simulink model "gm_tutorial1_1_mq"  (R2020b)
settings: Solver=FixedStepDiscrete  StartTime=0.0  StopTime=simulation_stop_time  RelTol=1e-3
undefined symbols (not defined in the file or in its folder): sample_time
libraries: simulink x1, modelsimlib x1
settings Model: Creator=yixingli  LastModifiedBy=harsh
settings DataIOCC: LimitDataPoints=on  SaveOutput=off  SignalLogging=off  SaveTime=off
settings OptimizationCC: BlockReduction=off  ConditionallyExecuteInputs=off  DefaultParameterBehavior=Inlined  ExpressionDepthLimit=2147483647  LifeSpan=inf
settings DebuggingCC: AlgebraicLoopMsg=error  UnderspecifiedInitializationDetection=Classic  MergeDetectMultiDrivingBlocksExec=none  InheritedTsInSrcMsg=none  SingleTaskRateTransMsg=error  ParameterPrecisionLossMsg=none  AllowSymbolicDim=off  StateNameClashWarn=warning  StrictBusMsg=ErrorOnBusTreatedAsVector  SFUnexpectedBacktrackingDiag=warning  SFNoUnconditionalDefaultTransitionDiag=warning  SFExecutionAtInitializationDiag=none  ArithmeticOperatorsInVariantConditions=warning
settings HardwareCC: ProdBitPerPointer=32  ProdBitPerSizeT=32  ProdBitPerPtrDiffT=32  ProdLargestAtomicFloat=None  ProdIntDivRoundTo=Undefined  ProdEndianess=Unspecified  ProdWordSize=32  ProdHWDeviceType=ASIC/FPGA->ASIC/FPGA  ProdEqTarget=off
settings SFSimCC: SimUseLocalCustomCode=off  CustomCodeUndefinedFunction=UseInterfaceOnly
settings RTWCC: RTWUseLocalCustomCode=off
settings CodeAppCC: StateflowObjectComments=on
settings GRTTargetCC: TargetLangStandard=C89/C90 (ANSI)
settings ConfigComp: CovScope=ReferencedModels  CovMetricSettings=dw  CovSaveCumulativeToWorkspaceVar=on  CovSaveSingleToWorkspaceVar=on  CovExternalEMLEnable=off  CovSFcnEnable=off

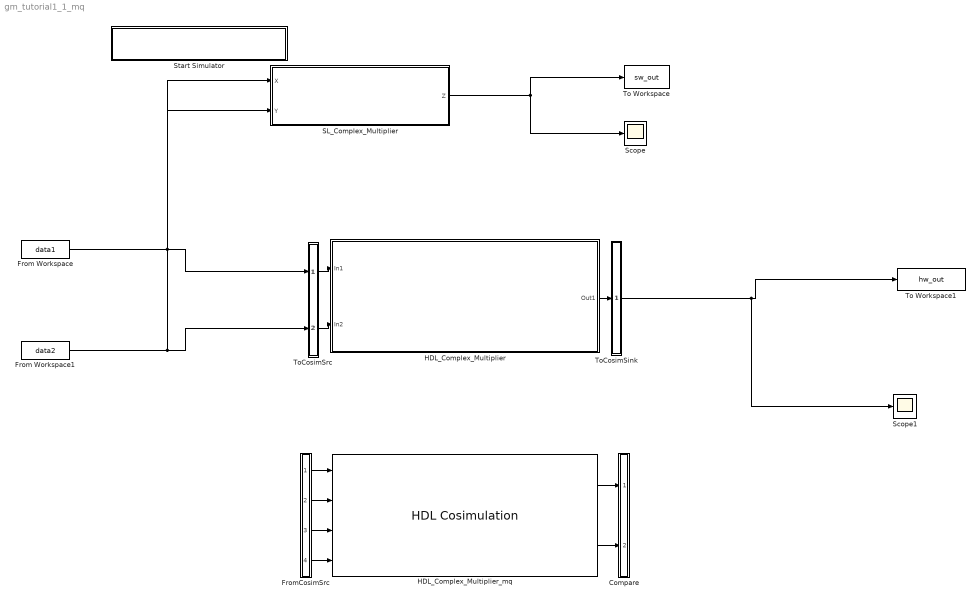
== system gm_tutorial1_1_mq ==
  Compare : Subsystem
      mask Display: disp('')
  From Workspace : FromWorkspace  VariableName=data1  SampleTime=sample_time  Interpolate=off  OutputAfterFinalValue=Setting to zero
  From Workspace1 : FromWorkspace  VariableName=data2  SampleTime=sample_time  Interpolate=off  OutputAfterFinalValue=Setting to zero
  FromCosimSrc : Subsystem
      mask Display: disp('')
  HDL_Complex_Multiplier : Subsystem
  HDL_Complex_Multiplier_mq : modelsimlib/HDL Cosimulation  PortPaths=/HDL_Complex_Multiplier/In1_re;/HDL_Complex_Multiplier/In1_im;/HDL_Complex_Multiplier/In2_re;/HDL_Complex_Multiplier/In2_im;/HDL_Complex_Multiplier/Out1_re;/HDL_Complex_Multiplier/Out1_im  PortModes=[1 1 1 1 2 2 ]  PortTimes=[-1 -1 -1 -1 9.9999999999999995474811182588625868561393872369080781936645507813e-07 9.9999999999999995474811182588625868561393872369080781936645507813e-07 ]  PortSigns=[-1 -1 -1 -1 1 1 ]  PortFracLengths=[0,0,0,0,16,16]  CommLocal=on  CommSharedMemory=on  CommPortNumber=4449  CommShowInfo=on  ClockModes=[]  ClockTimes=[]  TclPreSimCommand=|  TclPostSimCommand="puts \"done\""  TimingMode=ns  TimingScaleFactor=10000000  idxCellArray={'UNUSED_VAR'}  CosimBypass=Full Simulation  AllowDirectFeedthrough=on  ProductName=EDA Simulator Link MQ  RunAutoTimescale=off  HdlClocks=0  PreRunTime=40  PreRunTimeUnit=ns
      | puts "Running Simulink Cosimulation block.";
      |  puts "Chip Name: --> tutorial1_1/HDL_Complex_Multiplier";
      |  puts "Target language: --> verilog";
      |  puts "Target directory: --> hdl_prj\hdlsrc\tutorial1_1";
      |  puts [clock format [clock seconds]];
      | # Clock force command;
      | force /HDL_Complex_Multiplier/clk 0 0ns, 1 5ns -r 10ns;
      | # Clock enable force command;
      | force /HDL_Complex_Multiplier/clk_enable 0 0ns, 1 37ns;
      | # Reset force command;
      | force /HDL_Complex_Multiplier/reset 1 0ns, 0 27ns;
      settings: SourceProductBaseCode=ES
  SL_Complex_Multiplier : Subsystem
  Scope : Scope
  Scope1 : Scope
  Start Simulator : Subsystem
      settings: OpenFcn=|
      | try
      |    cosimDirName = pwd;
      |    cd 'hdl_prj\hdlsrc\tutorial1_1';
      |    vsim('tclstart',gm_tutorial1_1_mq_tcl);
      |    cd (cosimDirName);
      |    clear cosimDirName;
      | catch me
      |    disp('Failed to launch cosimulator with "vsim"');
      |    disp (me.message);
      |    cd (cosimDirName);
      |    clear cosimDirName;
      | end
      mask Display: disp(['vsimulink  -voptargs=+acc work.HDL_Complex_Multiplier' char(10) 'Double-click here to launch ModelSim'])
  To Workspace : ToWorkspace  VariableName=sw_out  SaveFormat=Structure With Time  SampleTime=-1
  To Workspace1 : ToWorkspace  VariableName=hw_out  SaveFormat=Structure With Time  SampleTime=-1
  ToCosimSink : Subsystem
      mask Display: disp('')
  ToCosimSrc : Subsystem
      mask Display: disp('')
  wires:
  SL_Complex_Multiplier/1(Z) -> To Workspace/1, Scope/1
  From Workspace/1 -> SL_Complex_Multiplier/1(X), ToCosimSrc/1(in1)
  From Workspace1/1 -> SL_Complex_Multiplier/2(Y), ToCosimSrc/2(in2)
  ToCosimSrc/1(out1) -> HDL_Complex_Multiplier/1(In1)
  ToCosimSrc/2(out2) -> HDL_Complex_Multiplier/2(In2)
  HDL_Complex_Multiplier/1(Out1) -> ToCosimSink/1(in1)
  ToCosimSink/1(out1) -> To Workspace1/1, Scope1/1
  FromCosimSrc/1(out1) -> HDL_Complex_Multiplier_mq/1
  FromCosimSrc/2(out2) -> HDL_Complex_Multiplier_mq/2
  FromCosimSrc/3(out3) -> HDL_Complex_Multiplier_mq/3
  FromCosimSrc/4(out4) -> HDL_Complex_Multiplier_mq/4
  HDL_Complex_Multiplier_mq/1 -> Compare/1(in1)
  HDL_Complex_Multiplier_mq/2 -> Compare/2(in2)

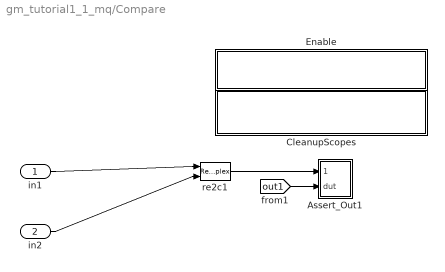
== system gm_tutorial1_1_mq/Compare ==
  in1 : Inport
  in2 : Inport  Port=2
  Assert_Out1 : Subsystem
  CleanupScopes : Subsystem
      settings: OpenFcn=|
      | blkName = gcb; %self block
      | idx = regexp(blkName, '/CleanupScopes$', 'once');
      | blkParent = blkName(1:idx-1);
      | blks=find_system(blkParent, 'LookUnderMasks', 'all','blocktype', 'Scope');
      | for itr = 1:length(blks)
      | 	 hScopeCfg = get_param(blks{itr},'ScopeConfiguration');
      | 	 hScopeCfg.Visible = ~ hScopeCfg.Visible;
      | end
      | drawnow;
      mask Display: fprintf(message('hdlcoder:cosim:vnl_dblclick').getString());
  Enable : Subsystem
      settings: OpenFcn=|
      | blkName = gcb;
      | idx = regexp(blkName, '/Enable$', 'once');
      | blkParent = blkName(1:idx-1);
      | blks=find_system(blkParent, 'LookUnderMasks', 'all','blocktype', 'Assertion');
      | e = get_param(blks{1}, 'Enabled');
      | if strcmp(e, 'on'), f= 'off';, else, f = 'on';, end
      | for ii=1:length(blks), set_param(blks{ii}, 'Enabled', f);, end
      | set_param(gcb, 'MaskDisplay',['fprintf(message(''hdlcoder:cosim:vnl_dblclick_assertions'',','''',upper(e),'''',').getString())']);
      mask Display: fprintf(message('hdlcoder:cosim:vnl_dblclick_assertions','OFF').getString());
  re2c1 : RealImagToComplex
  wires:
  in2/1 -> re2c1/2
  in1/1 -> re2c1/1
  re2c1/1 -> Assert_Out1/1(cosim)
  [out1] -> Assert_Out1/2(dut)

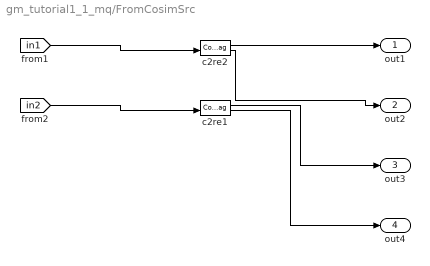
== system gm_tutorial1_1_mq/FromCosimSrc ==
  c2re1 : ComplexToRealImag
  c2re2 : ComplexToRealImag
  out1 : Outport
  out2 : Outport  Port=2
  out3 : Outport  Port=3
  out4 : Outport  Port=4
  wires:
  [in2] -> c2re1/1
  [in1] -> c2re2/1
  c2re2/1 -> out1/1
  c2re2/2 -> out2/1
  c2re1/1 -> out3/1
  c2re1/2 -> out4/1

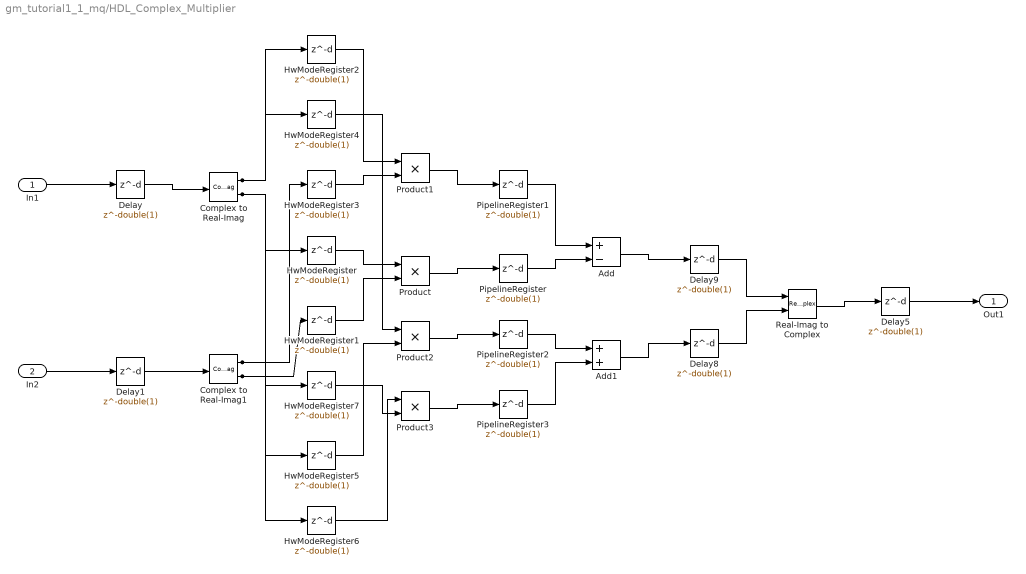
== system gm_tutorial1_1_mq/HDL_Complex_Multiplier ==
  In1 : Inport  OutDataTypeStr=fixdt(1, 12, 8)  PortDimensions=1  SampleTime=1e-06
      settings: SignalType=complex
  In2 : Inport  Port=2  OutDataTypeStr=fixdt(1, 12, 8)  PortDimensions=1  SampleTime=1e-06
      settings: SignalType=complex
  Add : Sum  Inputs=+-  AccumDataTypeStr=fixdt(1, 25, 16)  OutDataTypeStr=fixdt(1, 25, 16)  SampleTime=1e-06
  Add1 : Sum  AccumDataTypeStr=fixdt(1, 25, 16)  OutDataTypeStr=fixdt(1, 25, 16)  SampleTime=1e-06
  Complex to Real-Imag : ComplexToRealImag  SampleTime=1e-06
  Complex to Real-Imag1 : ComplexToRealImag  SampleTime=1e-06
  Delay{,1,5,8..9} (5 alike) : Delay  DelayLength=double(1)  InitialCondition=0  SampleTime=1e-06
  HwModeRegister{,1..7} (8 alike) : Delay  DelayLength=double(1)  InitialCondition=0  SampleTime=1e-06
  PipelineRegister{,1..3} (4 alike) : Delay  DelayLength=double(1)  InitialCondition=0  SampleTime=1e-06
  Product{,1..3} (4 alike) : Product  Inputs=**  OutDataTypeStr=fixdt(1, 24, 16)  SampleTime=1e-06
  Real-Imag to Complex : RealImagToComplex  ConstantPart="fi(0,1,25,16,\"hex\",\"0000000\")"  SampleTime=1e-06
  Out1 : Outport
  wires:
  HwModeRegister7/1 -> Product3/2
  HwModeRegister6/1 -> Product3/1
  Product3/1 -> PipelineRegister3/1
  HwModeRegister5/1 -> Product2/2
  HwModeRegister4/1 -> Product2/1
  Product2/1 -> PipelineRegister2/1
  HwModeRegister3/1 -> Product1/2
  HwModeRegister2/1 -> Product1/1
  Product1/1 -> PipelineRegister1/1
  HwModeRegister1/1 -> Product/2
  HwModeRegister/1 -> Product/1
  Product/1 -> PipelineRegister/1
  Real-Imag to Complex/1 -> Delay5/1
  PipelineRegister3/1 -> Add1/2
  PipelineRegister2/1 -> Add1/1
  PipelineRegister1/1 -> Add/1
  PipelineRegister/1 -> Add/2
  Delay9/1 -> Real-Imag to Complex/1
  Delay8/1 -> Real-Imag to Complex/2
  Delay5/1 -> Out1/1
  Delay1/1 -> Complex to Real-Imag1/1
  Delay/1 -> Complex to Real-Imag/1
  Complex to Real-Imag1/2 -> HwModeRegister5/1, HwModeRegister1/1
  Complex to Real-Imag1/1 -> HwModeRegister6/1, HwModeRegister3/1
  Complex to Real-Imag/2 -> HwModeRegister7/1, HwModeRegister/1
  Complex to Real-Imag/1 -> HwModeRegister4/1, HwModeRegister2/1
  Add1/1 -> Delay8/1
  Add/1 -> Delay9/1
  In2/1 -> Delay1/1
  In1/1 -> Delay/1

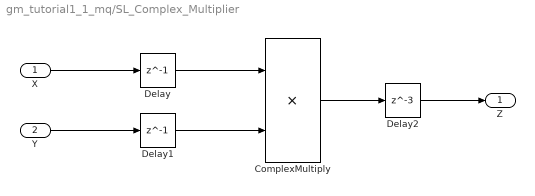
== system gm_tutorial1_1_mq/SL_Complex_Multiplier ==
  X : Inport
  Y : Inport  Port=2
  ComplexMultiply : Product
  Delay : Delay  DelayLength=1  InitialCondition=0
  Delay1 : Delay  DelayLength=1  InitialCondition=0
  Delay2 : Delay  DelayLength=3  InitialCondition=0
  Z : Outport  VectorParamsAs1DForOutWhenUnconnected=off
  wires:
  ComplexMultiply/1 -> Delay2/1
  X/1 -> Delay/1
  Y/1 -> Delay1/1
  Delay1/1 -> ComplexMultiply/2
  Delay/1 -> ComplexMultiply/1
  Delay2/1 -> Z/1

== system gm_tutorial1_1_mq/Start Simulator ==

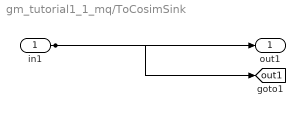
== system gm_tutorial1_1_mq/ToCosimSink ==
  in1 : Inport
  out1 : Outport
  tag scope: out1=global
  wires:
  in1/1 -> out1/1, [out1]

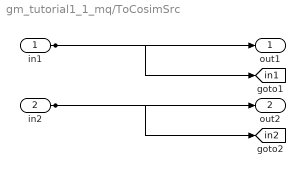
== system gm_tutorial1_1_mq/ToCosimSrc ==
  in1 : Inport
  in2 : Inport  Port=2
  out1 : Outport
  out2 : Outport  Port=2
  tag scope: in1=global, in2=global
  wires:
  in1/1 -> out1/1, [in1]
  in2/1 -> out2/1, [in2]

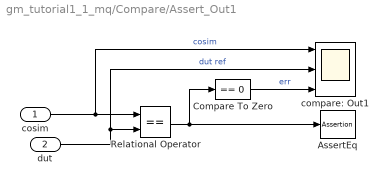
== system gm_tutorial1_1_mq/Compare/Assert_Out1 ==
  cosim : Inport
  dut : Inport  Port=2
  AssertEq : Assertion  StopWhenAssertionFail=off
  Compare To Zero : simulink/Logic and Bit Operations/Compare To Zero  relop===  OutDataTypeStr=boolean
  Relational Operator : RelationalOperator  Operator===  OutDataTypeStr=boolean  RndMeth=Nearest
  compare: Out1 : Scope  NumInputPorts=3
  wires:
  Compare To Zero/1 -> compare: Out1/3  "err"
  Relational Operator/1 -> Compare To Zero/1, AssertEq/1
  cosim/1 -> compare: Out1/1, Relational Operator/1  "cosim"
  dut/1 -> compare: Out1/2, Relational Operator/2  "dut ref"

== system gm_tutorial1_1_mq/Compare/CleanupScopes ==

== system gm_tutorial1_1_mq/Compare/Enable ==
